simulink model "Placement_pole"  (R2017a)
settings: Solver=VariableStepAuto  StartTime=0.0  StopTime=2000  RelTol=1e-3
settings Model: Creator=telep  LastModifiedBy=telep

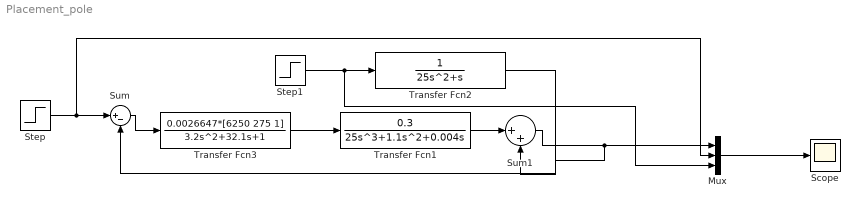
== system Placement_pole ==
  Mux : Mux  Inputs=3
  Scope : Scope
  Step : Step  SampleTime=0
  Step1 : Step  Time=1000  SampleTime=0
  Sum : Sum  Inputs=|+-
  Sum1 : Sum  Inputs=|++
  Transfer Fcn1 : TransferFcn  Numerator=[0.3]  Denominator=[25 1.1 0.004 0]
  Transfer Fcn2 : TransferFcn  Denominator=[25 1 0]
  Transfer Fcn3 : TransferFcn  Numerator=0.0026647*[6250 275 1]  Denominator=[3.2 32.1 1]
  wires:
  Step/1 -> Sum/1, Mux/2
  Mux/1 -> Scope/1
  Transfer Fcn3/1 -> Transfer Fcn1/1
  Sum/1 -> Transfer Fcn3/1
  Transfer Fcn1/1 -> Sum1/1
  Transfer Fcn2/1 -> Sum1/2
  Sum1/1 -> Sum/2, Mux/1
  Step1/1 -> Mux/3, Transfer Fcn2/1
